simulink model "flightControlSystem2"  (R2019a)
settings: Solver=ode3  StartTime=0  StopTime=TFinal  FixedStep=Ts  RelTol=1e-3  EnableMultiTasking=on
InitFcn:
  | %生成模板
  | temp_Image = uint8(ones(120,160));
  | 
  | [m,n] = size(temp_Image);
  | angle = 10*pi/180;
  | 
  | left_point = 70;
  | right_point = 90;
  | j = 71;
  | for i = 1:50
  |     temp_left_point = floor(left_point - i*sin(angle));
  |     temp_right_point = floor(right_point + i*sin(angle));
  |     if temp_left_point < 1
  |         temp_left_point = 1;
  |     end
  |     if temp_right_point > 180
  |         temp_right_point = 180;
  |     end
  |     temp_Image(j,temp_left_point:temp_right_point) = 0;
  |     j = j+1;
  | end
undefined symbols (not defined in the file): codertarget, Controller, DiscIntNeverNeededParam, Discrete, Estimator, g, gray, init, pos_ref, Sensors, takeoff_flag, Time, Ts, Vehicle
libraries: simulink x60, visiontransforms x4, sharedtransform x3, ctrlSharedLib x2, visionsinks x2, sharedutil x1, visionanalysis x1, parrotlib x1
(part 1 of 3)
settings Model: ExtModeTrigDuration=80  Creator=The MathWorks, Inc.  LastModifiedBy=Sharlene
settings DataIOCC: LimitDataPoints=on  SaveFormat=StructureWithTime  SaveOutput=off  DSMLogging=off  SaveTime=off  ReturnWorkspaceOutputs=off
settings OptimizationCC: BlockReduction=off  EnhancedBackFolding=on  PassReuseOutputArgsAs=Individual arguments  MaxStackSize=64  OptimizeBlockOrder=speed  DifferentSizesBufferReuse=on  OptimizationCustomize=off
settings DebuggingCC: AlgebraicLoopMsg=none  ParameterPrecisionLossMsg=none  ParameterTunabilityLossMsg=error  UnconnectedInputMsg=none  UnconnectedOutputMsg=none  UnconnectedLineMsg=none  BusObjectLabelMismatch=error  PregeneratedLibrarySubsystemCodeDiagnostic=none  SFUnexpectedBacktrackingDiag=warning  SFNoUnconditionalDefaultTransitionDiag=warning  SFExecutionAtInitializationDiag=none  ArithmeticOperatorsInVariantConditions=warning
settings HardwareCC: ProdBitPerPointer=32  ProdBitPerSizeT=32  ProdBitPerPtrDiffT=32  ProdLargestAtomicInteger=Long  ProdWordSize=32  ProdHWDeviceType=ARM Compatible->ARM 9  UseEmbeddedCoderFeatures=off  UseSimulinkCoderFeatures=off
settings ModelReferenceCC: ModelReferenceNumInstancesAllowed=Single  PropagateSignalLabelsOutOfModel=off
settings SFSimCC: SimUseLocalCustomCode=off  MATLABDynamicMemAlloc=off
settings RTWCC: SystemTargetFile=ert.tlc  HardwareBoard=PARROT Mambo  TLCOptions=-aInlineSetEventsForThisBaseRateFcn=TLC_FALSE -aSuppressMultiTaskScheduler=TLC_FALSE -aRateBasedStepFcn=1  TemplateMakefile=ert_default_tmf  RTWUseLocalCustomCode=off  Toolchain=Sourcery G++ Lite GNU Toolchain for Drones  IncludeHyperlinkInReport=on
settings CodeAppCC: ForceParamTrailComments=on  IgnoreCustomStorageClasses=off  MaxIdLength=63  OperatorAnnotations=on  SimulinkDataObjDesc=on  SFDataObjDesc=on  InsertBlockDesc=on
settings ERTTargetCC: CombineOutputUpdateFcns=off  SupportNonInlinedSFcns=on
settings ConfigComp: CovMetricSettings=dw  CovHtmlReporting=on  CovSaveCumulativeToWorkspaceVar=on  CovSaveSingleToWorkspaceVar=on  CovExternalEMLEnable=off  CovSFcnEnable=off

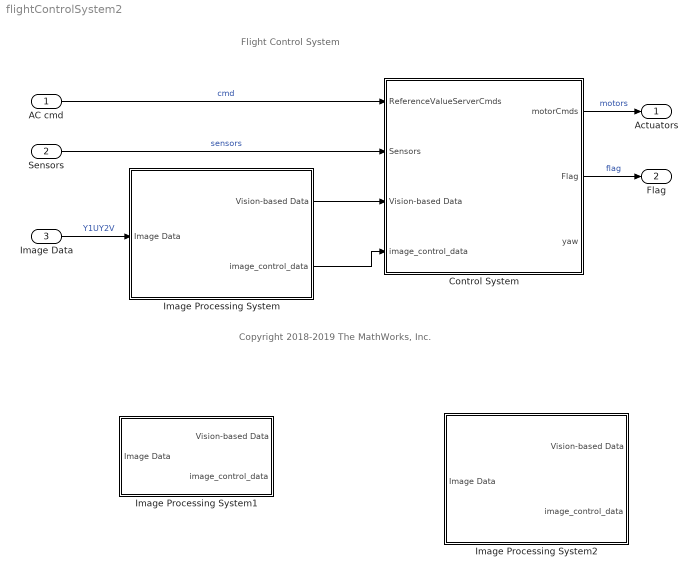
== system flightControlSystem2 ==
  note: Copyright 2018-2019 The MathWorks, Inc.
  note: Flight Control System
  AC cmd : Inport  OutDataTypeStr=Bus: CommandBus  BusOutputAsStruct=on
  Sensors : Inport  Port=2  OutDataTypeStr=Bus: SensorsBus  BusOutputAsStruct=on
  Image Data : Inport  Tag=IP_IN  InitFcn=codertarget.parrot.internal.inportCallback(gcb);  Port=3  OutDataTypeStr=uint8  PortDimensions=[4 9600]  BusOutputAsStruct=on
  Control System : Subsystem  InitFcn=codertarget.parrot.internal.fcsSubsystemCallback(gcb);  TreatAsAtomicUnit=on  SystemSampleTime=Ts
  Image Processing System : Subsystem  Tag=IP_SUB  InitFcn=codertarget.parrot.internal.ipSubsystemCallback(gcb);  TreatAsAtomicUnit=on  SystemSampleTime=40*Ts  RTWFcnName=ImageFunction
      settings: RTWSystemCode=Inline  RTWFcnNameOpts=User specified
  Image Processing System1 : Subsystem  Tag=IP_SUB  InitFcn=codertarget.parrot.internal.ipSubsystemCallback(gcb);  TreatAsAtomicUnit=on  SystemSampleTime=40*Ts  RTWFcnName=ImageFunction
      settings: RTWSystemCode=Inline  RTWFcnNameOpts=User specified
  Image Processing System2 : Subsystem  Tag=IP_SUB  InitFcn=codertarget.parrot.internal.ipSubsystemCallback(gcb);  TreatAsAtomicUnit=on  SystemSampleTime=40*Ts  RTWFcnName=ImageFunction
      settings: RTWSystemCode=Inline  RTWFcnNameOpts=User specified
  Actuators : Outport  OutDataTypeStr=single  PortDimensions=4
  Flag : Outport  Port=2  OutDataTypeStr=uint8  PortDimensions=1
  wires:
  AC cmd/1 -> Control System/1(ReferenceValueServerCmds)  "cmd"
  Control System/1(motorCmds) -> Actuators/1  "motors"
  Sensors/1 -> Control System/2(Sensors)  "sensors"
  Control System/2(Flag) -> Flag/1  "flag"
  Image Data/1 -> Image Processing System/1(Image Data)  "Y1UY2V"
  Image Processing System/1(Vision-based Data) -> Control System/3(Vision-based Data)
  Image Processing System/2(image_control_data) -> Control System/4("image_control_data ")

== system flightControlSystem2/Control System ==
  note: Position or Orientation Control
  note: Use this subsystem to change the path of the
      | Minidrone depending on the input Vision-based
      | Data
  note: Derived from the work by Sertac
      | Karaman and Fabian Riether
  ReferenceValueServerCmds : Inport  OutDataTypeStr=Bus: CommandBus
  Sensors : Inport  Port=2  OutDataTypeStr=Bus: SensorsBus  BusOutputAsStruct=on
  Vision-based Data : Inport  Port=3
  "image_control_data " : Inport  Port=4
  Bus Selector1 : BusSelector  OutputSignals=opticalFlow_data
  Bus Selector4 : BusSelector  OutputSignals=VisionSensors,SensorCalibration
  Control Mode Update : BusAssignment  AssignedSignals=controlModePosVSOrient
  Controller : Subsystem
  Crash Predictor Flags : Subsystem
  Path Planning : Subsystem
  Path Planning1 : Subsystem
  Path Planning2 : Subsystem
  State Estimator : Subsystem
  To Workspace : ToWorkspace  VariableName=estimatedStates  SaveFormat=Structure With Time  SampleTime=-1
  controlModePosVsOrient : Constant  OutDataTypeStr=boolean
  motorCmds : Outport
  Flag : Outport  Port=2
  yaw : Outport  Port=3
  wires:
  ReferenceValueServerCmds/1 -> Control Mode Update/1
  Bus Selector1/1 -> State Estimator/3(opticalFlow_datin)  "<opticalFlow_data>"
  Bus Selector4/2 -> State Estimator/4(sensorCalibration_datin)  "<SensorCalibration>"
  Path Planning/1(UpdatedReferenceCmds) -> Controller/1(ReferenceValueServerBus)
  Bus Selector4/1 -> Bus Selector1/1  "<VisionSensors>"
  Vision-based Data/1 -> Path Planning/3(drone_xyz)
  Crash Predictor Flags/1(Flag) -> Flag/1
  Control Mode Update/1 -> Path Planning/1(ReferenceValueServerCmds)
  controlModePosVsOrient/1 -> Control Mode Update/2, State Estimator/1(controlModePosVSOrient_flagin)
  Controller/1(motors_refout) -> motorCmds/1
  Sensors/1 -> State Estimator/2(sensor_data_in), Crash Predictor Flags/3(Sensors), Bus Selector4/1
  State Estimator/1(states_estim) -> Crash Predictor Flags/1(states_estim), To Workspace/1, Controller/2(states_estim)
  State Estimator/2(Alt_prs) -> Crash Predictor Flags/2(Alt_prs)
  Controller/2(yaw) -> Path Planning/4(yaw), yaw/1
  "image_control_data "/1 -> Path Planning/2(image_control_data)

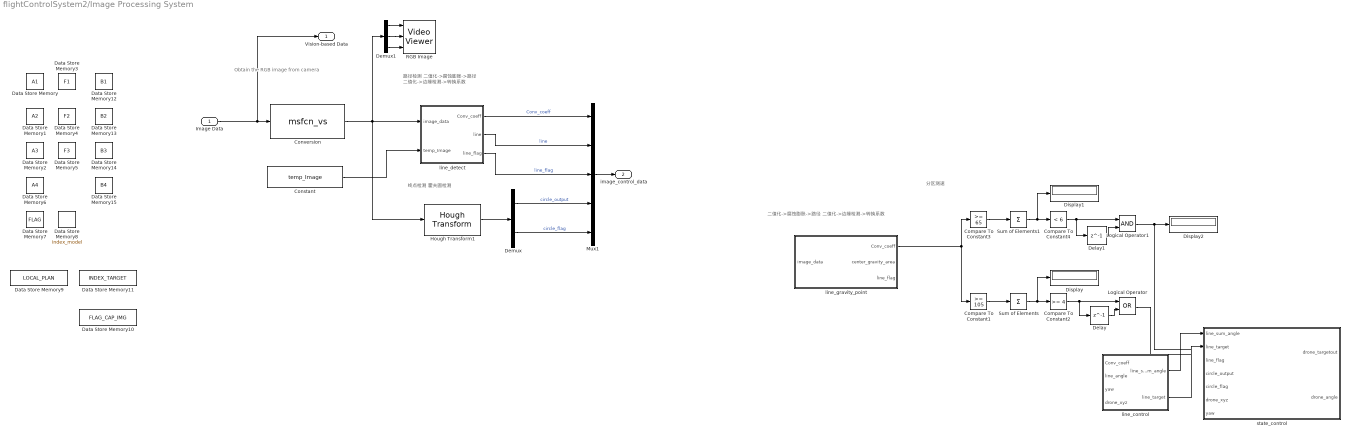
== system flightControlSystem2/Image Processing System ==
  note: 二值化->腐蚀膨胀->路径
      | 二值化->边缘检测->转换系数
  note: 终点检测
      | 霍夫圆检测
  note: Obtain the RGB image from camera
  note: 路径检测
      | 二值化->腐蚀膨胀->路径
      | 二值化->边缘检测->转换系数
  note: 分区测速
  Image Data : Inport
  Compare To Constant1 : simulink/Logic and Bit Operations/Compare To Constant  relop=>=  const=105  OutDataTypeStr=boolean
  Compare To Constant2 : simulink/Logic and Bit Operations/Compare To Constant  relop=>=  const=4  OutDataTypeStr=boolean
  Compare To Constant3 : simulink/Logic and Bit Operations/Compare To Constant  relop=>=  const=65  OutDataTypeStr=boolean
  Compare To Constant4 : simulink/Logic and Bit Operations/Compare To Constant  relop=<  const=6  OutDataTypeStr=boolean
  Constant : Constant  Value=temp_Image
  Conversion : M-S-Function  FunctionName=msfcn_vs
      mask Display: disp('PARROT Image Conversion')
  Data Store Memory : DataStoreMemory  DataStoreName=A1  ReadBeforeWriteMsg=warning  WriteAfterWriteMsg=warning  WriteAfterReadMsg=warning  ShowAdditionalParam=off  OutDataTypeStr=double
  Data Store Memory1 : DataStoreMemory  DataStoreName=A2  ReadBeforeWriteMsg=warning  WriteAfterWriteMsg=warning  WriteAfterReadMsg=warning  ShowAdditionalParam=off  OutDataTypeStr=double
  Data Store Memory10 : DataStoreMemory  DataStoreName=FLAG_CAP_IMG  ReadBeforeWriteMsg=warning  WriteAfterWriteMsg=warning  WriteAfterReadMsg=warning  InitialValue=1  ShowAdditionalParam=off  OutDataTypeStr=double
  Data Store Memory11 : DataStoreMemory  DataStoreName=INDEX_TARGET  ReadBeforeWriteMsg=warning  WriteAfterWriteMsg=warning  WriteAfterReadMsg=warning  InitialValue=1  ShowAdditionalParam=off  OutDataTypeStr=double
  Data Store Memory12 : DataStoreMemory  DataStoreName=B1  ReadBeforeWriteMsg=warning  WriteAfterWriteMsg=warning  WriteAfterReadMsg=warning  ShowAdditionalParam=off  OutDataTypeStr=double
  Data Store Memory13 : DataStoreMemory  DataStoreName=B2  ReadBeforeWriteMsg=warning  WriteAfterWriteMsg=warning  WriteAfterReadMsg=warning  ShowAdditionalParam=off  OutDataTypeStr=double
  Data Store Memory14 : DataStoreMemory  DataStoreName=B3  ReadBeforeWriteMsg=warning  WriteAfterWriteMsg=warning  WriteAfterReadMsg=warning  ShowAdditionalParam=off  OutDataTypeStr=double
  Data Store Memory15 : DataStoreMemory  DataStoreName=B4  ReadBeforeWriteMsg=warning  WriteAfterWriteMsg=warning  WriteAfterReadMsg=warning  ShowAdditionalParam=off  OutDataTypeStr=double
  Data Store Memory2 : DataStoreMemory  DataStoreName=A3  ReadBeforeWriteMsg=warning  WriteAfterWriteMsg=warning  WriteAfterReadMsg=warning  ShowAdditionalParam=off  OutDataTypeStr=double
  Data Store Memory3 : DataStoreMemory  DataStoreName=F1  ReadBeforeWriteMsg=warning  WriteAfterWriteMsg=warning  WriteAfterReadMsg=warning  ShowAdditionalParam=off  OutDataTypeStr=double
  Data Store Memory4 : DataStoreMemory  DataStoreName=F2  ReadBeforeWriteMsg=warning  WriteAfterWriteMsg=warning  WriteAfterReadMsg=warning  ShowAdditionalParam=off  OutDataTypeStr=double
  Data Store Memory5 : DataStoreMemory  DataStoreName=F3  ReadBeforeWriteMsg=warning  WriteAfterWriteMsg=warning  WriteAfterReadMsg=warning  InitialValue=[0;0;0]  ShowAdditionalParam=off  OutDataTypeStr=double
  Data Store Memory6 : DataStoreMemory  DataStoreName=A4  ReadBeforeWriteMsg=warning  WriteAfterWriteMsg=warning  WriteAfterReadMsg=warning  ShowAdditionalParam=off  OutDataTypeStr=double
  Data Store Memory7 : DataStoreMemory  DataStoreName=FLAG  ReadBeforeWriteMsg=warning  WriteAfterWriteMsg=warning  WriteAfterReadMsg=warning  ShowAdditionalParam=off  OutDataTypeStr=double
  Data Store Memory8 : DataStoreMemory  DataStoreName=index_model  ReadBeforeWriteMsg=warning  WriteAfterWriteMsg=warning  WriteAfterReadMsg=warning  InitialValue=1  ShowAdditionalParam=off  OutDataTypeStr=double
  Data Store Memory9 : DataStoreMemory  DataStoreName=LOCAL_PLAN  ReadBeforeWriteMsg=warning  WriteAfterWriteMsg=warning  WriteAfterReadMsg=warning  InitialValue=ones(10,2)  ShowAdditionalParam=off  OutDataTypeStr=double
  Delay : Delay  DelayLength=1  InitialCondition=0
  Delay1 : Delay  DelayLength=1  InitialCondition=0
  Demux : Demux  Outputs=2
  Demux1 : Demux  Outputs=3
  Display : Display
  Display1 : Display
  Display2 : Display
  Hough Transform1 : visiontransforms/Hough Transform  theta_res=pi/180  rho_res=1  out_theta_rho=off  outdtmode=double  roundingMode=Nearest  overflowMode=on  firstCoeffMode=Binary point scaling  firstCoeffWordLength=16  firstCoeffFracLength=14  firstCoeffSlope=2^-14  secondCoeffMode=Binary point scaling  secondCoeffWordLength=32  secondCoeffFracLength=16  secondCoeffSlope=2^-16  prodOutputMode=Binary point scaling  prodOutputWordLength=32  prodOutputFracLength=20  prodOutputSlope=2^-20  accumMode=Binary point scaling  accumWordLength=32  accumFracLength=20  accumSlope=2^-20  outputMode=Binary point scaling  outputWordLength=16  outputFracLength=0  outputSlope=2^0  memoryMode=Binary point scaling  memoryWordLength=32  memoryFracLength=16  memorySlope=2^-16
      settings: SourceProductName=Computer Vision Toolbox  SourceProductBaseCode=VP
  Logical Operator : Logic  Operator=OR  AllPortsSameDT=off  OutDataTypeStr=boolean
  Logical Operator1 : Logic  AllPortsSameDT=off  OutDataTypeStr=boolean
  Mux1 : Mux  Inputs=5
  RGB Image : VideoViewer  imagePorts=separate color signals  FigPos=[238 767 414 175]
  Sum of Elements : Sum  Inputs=+  OutDataTypeStr=int8
  Sum of Elements1 : Sum  Inputs=+  OutDataTypeStr=int8
  line_control : MATLAB Function  TreatAsAtomicUnit=on
  line_detect : MATLAB Function  TreatAsAtomicUnit=on
  line_gravity_point : MATLAB Function  TreatAsAtomicUnit=on
  state_control : MATLAB Function  TreatAsAtomicUnit=on
  Vision-based Data : Outport
  image_control_data : Outport  Port=2
  wires:
  Image Data/1 -> Vision-based Data/1, Conversion/1
  Constant/1 -> line_detect/2(temp_Image)
  line_control/1(line_sum_angle) -> state_control/1(line_sum_angle)
  line_control/2(line_target) -> state_control/2(line_target)
  Sum of Elements1/1 -> Compare To Constant4/1, Display1/1
  Compare To Constant4/1 -> Delay1/1, Logical Operator1/1
  Compare To Constant3/1 -> Sum of Elements1/1
  Delay/1 -> Logical Operator/2
  Compare To Constant2/1 -> Logical Operator/1, Delay/1
  Logical Operator1/1 -> Display2/1
  Sum of Elements/1 -> Compare To Constant2/1, Display/1
  line_gravity_point/1(Conv_coeff) -> Compare To Constant1/1, Compare To Constant3/1
  Logical Operator/1 -> ?
  Compare To Constant1/1 -> Sum of Elements/1
  Delay1/1 -> Logical Operator1/2
  Conversion/1 -> line_detect/1(image_data), Hough Transform1/1, Demux1/1
  Demux/1 -> Mux1/4  "circle_output"
  line_detect/3(line_flag) -> Mux1/3  "line_flag"
  line_detect/1(Conv_coeff) -> Mux1/1  "Conv_coeff"
  Mux1/1 -> image_control_data/1
  Demux/2 -> Mux1/5  "circle_flag"
  Hough Transform1/1 -> Demux/1
  line_detect/2(line) -> Mux1/2  "line"
  Demux1/1 -> RGB Image/1
  Demux1/2 -> RGB Image/2
  Demux1/3 -> RGB Image/3

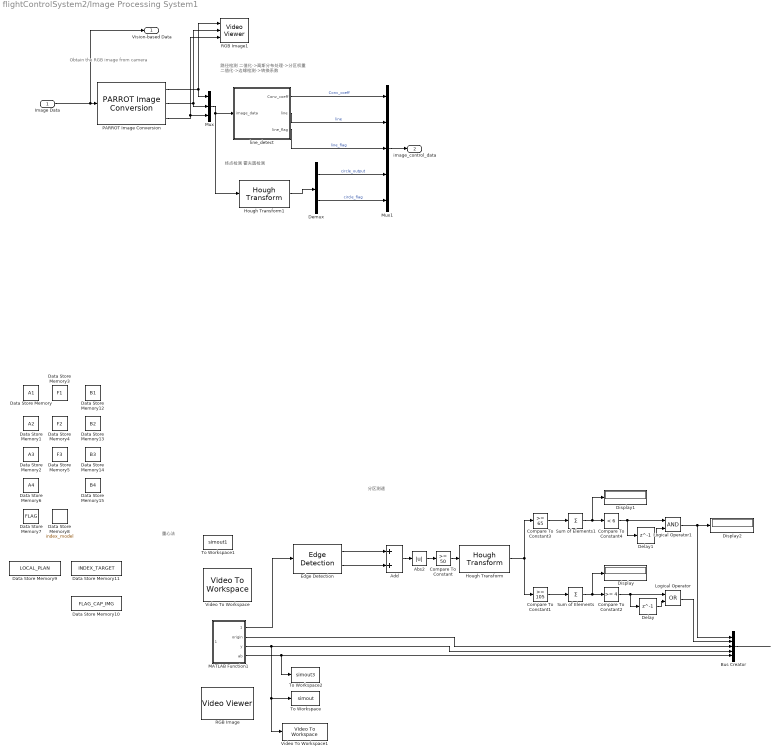
== system flightControlSystem2/Image Processing System1 ==
  note: 分区测速
  note: 重心法
  note: 路径检测
      | 二值化->高斯分布处理->分区权重
      | 二值化->边缘检测->转换系数
  note: 终点检测
      | 霍夫圆检测
  note: Obtain the RGB image from camera
  Image Data : Inport
  Abs2 : Abs
  Add : Sum
  Bus Creator : BusCreator  Inputs=5
  Compare To Constant : simulink/Logic and Bit Operations/Compare To Constant  relop=>=  const=50  OutDataTypeStr=boolean
  Compare To Constant1 : simulink/Logic and Bit Operations/Compare To Constant  relop=>=  const=105  OutDataTypeStr=boolean
  Compare To Constant2 : simulink/Logic and Bit Operations/Compare To Constant  relop=>=  const=4  OutDataTypeStr=boolean
  Compare To Constant3 : simulink/Logic and Bit Operations/Compare To Constant  relop=>=  const=65  OutDataTypeStr=boolean
  Compare To Constant4 : simulink/Logic and Bit Operations/Compare To Constant  relop=<  const=6  OutDataTypeStr=boolean
  Data Store Memory : DataStoreMemory  DataStoreName=A1  ReadBeforeWriteMsg=warning  WriteAfterWriteMsg=warning  WriteAfterReadMsg=warning  ShowAdditionalParam=off  OutDataTypeStr=double
  Data Store Memory1 : DataStoreMemory  DataStoreName=A2  ReadBeforeWriteMsg=warning  WriteAfterWriteMsg=warning  WriteAfterReadMsg=warning  ShowAdditionalParam=off  OutDataTypeStr=double
  Data Store Memory10 : DataStoreMemory  DataStoreName=FLAG_CAP_IMG  ReadBeforeWriteMsg=warning  WriteAfterWriteMsg=warning  WriteAfterReadMsg=warning  InitialValue=1  ShowAdditionalParam=off  OutDataTypeStr=double
  Data Store Memory11 : DataStoreMemory  DataStoreName=INDEX_TARGET  ReadBeforeWriteMsg=warning  WriteAfterWriteMsg=warning  WriteAfterReadMsg=warning  InitialValue=1  ShowAdditionalParam=off  OutDataTypeStr=double
  Data Store Memory12 : DataStoreMemory  DataStoreName=B1  ReadBeforeWriteMsg=warning  WriteAfterWriteMsg=warning  WriteAfterReadMsg=warning  ShowAdditionalParam=off  OutDataTypeStr=double
  Data Store Memory13 : DataStoreMemory  DataStoreName=B2  ReadBeforeWriteMsg=warning  WriteAfterWriteMsg=warning  WriteAfterReadMsg=warning  ShowAdditionalParam=off  OutDataTypeStr=double
  Data Store Memory14 : DataStoreMemory  DataStoreName=B3  ReadBeforeWriteMsg=warning  WriteAfterWriteMsg=warning  WriteAfterReadMsg=warning  ShowAdditionalParam=off  OutDataTypeStr=double
  Data Store Memory15 : DataStoreMemory  DataStoreName=B4  ReadBeforeWriteMsg=warning  WriteAfterWriteMsg=warning  WriteAfterReadMsg=warning  ShowAdditionalParam=off  OutDataTypeStr=double
  Data Store Memory2 : DataStoreMemory  DataStoreName=A3  ReadBeforeWriteMsg=warning  WriteAfterWriteMsg=warning  WriteAfterReadMsg=warning  ShowAdditionalParam=off  OutDataTypeStr=double
  Data Store Memory3 : DataStoreMemory  DataStoreName=F1  ReadBeforeWriteMsg=warning  WriteAfterWriteMsg=warning  WriteAfterReadMsg=warning  ShowAdditionalParam=off  OutDataTypeStr=double
  Data Store Memory4 : DataStoreMemory  DataStoreName=F2  ReadBeforeWriteMsg=warning  WriteAfterWriteMsg=warning  WriteAfterReadMsg=warning  ShowAdditionalParam=off  OutDataTypeStr=double
  Data Store Memory5 : DataStoreMemory  DataStoreName=F3  ReadBeforeWriteMsg=warning  WriteAfterWriteMsg=warning  WriteAfterReadMsg=warning  InitialValue=[0;0;0]  ShowAdditionalParam=off  OutDataTypeStr=double
  Data Store Memory6 : DataStoreMemory  DataStoreName=A4  ReadBeforeWriteMsg=warning  WriteAfterWriteMsg=warning  WriteAfterReadMsg=warning  ShowAdditionalParam=off  OutDataTypeStr=double
  Data Store Memory7 : DataStoreMemory  DataStoreName=FLAG  ReadBeforeWriteMsg=warning  WriteAfterWriteMsg=warning  WriteAfterReadMsg=warning  ShowAdditionalParam=off  OutDataTypeStr=double
  Data Store Memory8 : DataStoreMemory  DataStoreName=index_model  ReadBeforeWriteMsg=warning  WriteAfterWriteMsg=warning  WriteAfterReadMsg=warning  InitialValue=1  ShowAdditionalParam=off  OutDataTypeStr=double
  Data Store Memory9 : DataStoreMemory  DataStoreName=LOCAL_PLAN  ReadBeforeWriteMsg=warning  WriteAfterWriteMsg=warning  WriteAfterReadMsg=warning  InitialValue=ones(10,2)  ShowAdditionalParam=off  OutDataTypeStr=double
  Delay : Delay  DelayLength=1  InitialCondition=0
  Delay1 : Delay  DelayLength=1  InitialCondition=0
  Demux : Demux  Outputs=2
  Display : Display
  Display1 : Display
  Display2 : Display
  Edge Detection : visionanalysis/Edge Detection  method=Sobel  outputType=Gradient components  userDefinedThreshold=off  thresholdSource=Input port  threshold=20  thresholdTuning=4  edgeThinning=off  threshold_canny=[0.25 0.60]  autoPercent=70  sigma=1  roundingMode=Floor  overflowMode=off  prodOutputMode=Binary point scaling  prodOutputWordLength=32  prodOutputFracLength=8  prodOutputSlope=2^-8  accumSlope=2^-8  outputSlope=2^-4
      settings: SourceProductName=Computer Vision Toolbox  SourceProductBaseCode=VP
  Hough Transform : visiontransforms/Hough Transform  theta_res=pi/180  rho_res=1  out_theta_rho=off  outdtmode=double  roundingMode=Nearest  overflowMode=on  firstCoeffMode=Binary point scaling  firstCoeffWordLength=16  firstCoeffFracLength=14  firstCoeffSlope=2^-14  secondCoeffMode=Binary point scaling  secondCoeffWordLength=32  secondCoeffFracLength=16  secondCoeffSlope=2^-16  prodOutputMode=Binary point scaling  prodOutputWordLength=32  prodOutputFracLength=20  prodOutputSlope=2^-20  accumMode=Binary point scaling  accumWordLength=32  accumFracLength=20  accumSlope=2^-20  outputMode=Binary point scaling  outputWordLength=16  outputFracLength=0  outputSlope=2^0  memoryMode=Binary point scaling  memoryWordLength=32  memoryFracLength=16  memorySlope=2^-16
      settings: SourceProductName=Computer Vision Toolbox  SourceProductBaseCode=VP
  Hough Transform1 : visiontransforms/Hough Transform  theta_res=pi/180  rho_res=1  out_theta_rho=off  outdtmode=double  roundingMode=Nearest  overflowMode=on  firstCoeffMode=Binary point scaling  firstCoeffWordLength=16  firstCoeffFracLength=14  firstCoeffSlope=2^-14  secondCoeffMode=Binary point scaling  secondCoeffWordLength=32  secondCoeffFracLength=16  secondCoeffSlope=2^-16  prodOutputMode=Binary point scaling  prodOutputWordLength=32  prodOutputFracLength=20  prodOutputSlope=2^-20  accumMode=Binary point scaling  accumWordLength=32  accumFracLength=20  accumSlope=2^-20  outputMode=Binary point scaling  outputWordLength=16  outputFracLength=0  outputSlope=2^0  memoryMode=Binary point scaling  memoryWordLength=32  memoryFracLength=16  memorySlope=2^-16
      settings: SourceProductName=Computer Vision Toolbox  SourceProductBaseCode=VP
  Logical Operator : Logic  Operator=OR  AllPortsSameDT=off  OutDataTypeStr=boolean
  Logical Operator1 : Logic  AllPortsSameDT=off  OutDataTypeStr=boolean
  MATLAB Function1 : MATLAB Function  TreatAsAtomicUnit=on
  Mux : Mux  Inputs=3
  Mux1 : Mux  Inputs=5
  PARROT Image Conversion : parrotlib/PARROT Image Conversion  ImageFormat=RGB  R=on  Y=on  G=on  U=on  B=on  V=on
      settings: SourceProductName=Simulink Support Package for PARROT Minidrones
  RGB Image : VideoViewer  imagePorts=separate color signals  colormapValue=gray(256)  FigPos=[980.636363636364 356.545454545455 317.090909090909 234.909090909091]
  RGB Image1 : VideoViewer  imagePorts=separate color signals  FigPos=[238 767 414 175]
  Sum of Elements : Sum  Inputs=+  OutDataTypeStr=int8
  Sum of Elements1 : Sum  Inputs=+  OutDataTypeStr=int8
  To Workspace : ToWorkspace  VariableName=simout  SaveFormat=Timeseries  SampleTime=-1
  To Workspace1 : ToWorkspace  VariableName=simout1  SaveFormat=Timeseries  SampleTime=-1
  To Workspace2 : ToWorkspace  VariableName=simout3  SaveFormat=Timeseries  SampleTime=-1
  Video To Workspace : visionsinks/Video To Workspace  VariableName=RI  NumInputs=1  DataLimit=1  DecimationFactor=1  LogFi=off  InPortLabels=R|G|B
      settings: SourceProductName=Computer Vision Toolbox  SourceProductBaseCode=VP
  Video To Workspace1 : visionsinks/Video To Workspace  VariableName=RI2  NumInputs=1  DataLimit=1  DecimationFactor=1  LogFi=off  InPortLabels=R|G|B
      settings: SourceProductName=Computer Vision Toolbox  SourceProductBaseCode=VP
  line_detect : MATLAB Function  TreatAsAtomicUnit=on
  Vision-based Data : Outport
  image_control_data : Outport  Port=2
  wires:
  ? -> MATLAB Function1/1(R_Matrix), To Workspace1/1, Video To Workspace/1, RGB Image/1
  Sum of Elements1/1 -> Compare To Constant4/1, Display1/1
  Compare To Constant4/1 -> Delay1/1, Logical Operator1/1
  Compare To Constant3/1 -> Sum of Elements1/1
  Delay/1 -> Logical Operator/2
  Edge Detection/2 -> Add/2
  MATLAB Function1/1(R_stright) -> Edge Detection/1
  Compare To Constant2/1 -> Logical Operator/1, Delay/1
  Logical Operator1/1 -> Bus Creator/1, Display2/1
  Sum of Elements/1 -> Compare To Constant2/1, Display/1
  Compare To Constant1/1 -> Sum of Elements/1
  Edge Detection/1 -> Add/1
  Abs2/1 -> Compare To Constant/1
  Add/1 -> Abs2/1
  ? -> RGB Image/2
  ? -> RGB Image/3
  Bus Creator/1 -> ?
  MATLAB Function1/2(origin) -> Bus Creator/3
  MATLAB Function1/3(y) -> Bus Creator/4, To Workspace/1, Video To Workspace1/1
  Hough Transform/1 -> Compare To Constant1/1, Compare To Constant3/1
  MATLAB Function1/4(ab) -> Bus Creator/5, To Workspace2/1
  Compare To Constant/1 -> Hough Transform/1
  Logical Operator/1 -> Bus Creator/2
  Delay1/1 -> Logical Operator1/2
  Hough Transform1/1 -> Demux/1
  Demux/2 -> Mux1/5  "circle_flag"
  Image Data/1 -> Vision-based Data/1, PARROT Image Conversion/1
  PARROT Image Conversion/2 -> RGB Image1/2, Mux/2
  PARROT Image Conversion/3 -> RGB Image1/3, Mux/3
  line_detect/2(line) -> Mux1/2  "line"
  line_detect/1(Conv_coeff) -> Mux1/1  "Conv_coeff"
  line_detect/3(line_flag) -> Mux1/3  "line_flag"
  PARROT Image Conversion/1 -> RGB Image1/1, Mux/1
  Demux/1 -> Mux1/4  "circle_output"
  Mux/1 -> Hough Transform1/1, line_detect/1(image_data)
  Mux1/1 -> image_control_data/1

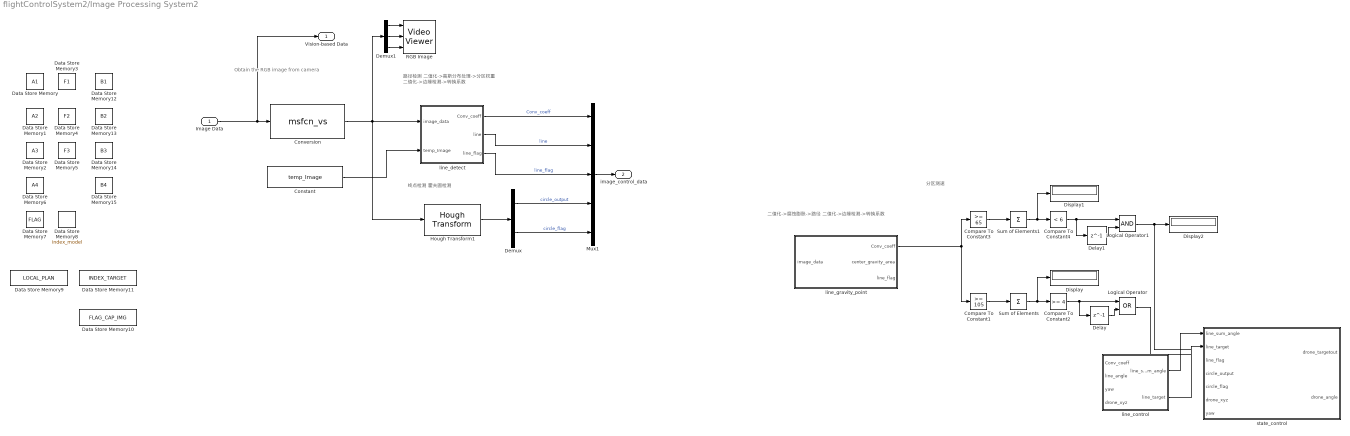
== system flightControlSystem2/Image Processing System2 ==
  note: 二值化->腐蚀膨胀->路径
      | 二值化->边缘检测->转换系数
  note: 终点检测
      | 霍夫圆检测
  note: Obtain the RGB image from camera
  note: 路径检测
      | 二值化->高斯分布处理->分区权重
      | 二值化->边缘检测->转换系数
  note: 分区测速
  Image Data : Inport
  Compare To Constant1 : simulink/Logic and Bit Operations/Compare To Constant  relop=>=  const=105  OutDataTypeStr=boolean
  Compare To Constant2 : simulink/Logic and Bit Operations/Compare To Constant  relop=>=  const=4  OutDataTypeStr=boolean
  Compare To Constant3 : simulink/Logic and Bit Operations/Compare To Constant  relop=>=  const=65  OutDataTypeStr=boolean
  Compare To Constant4 : simulink/Logic and Bit Operations/Compare To Constant  relop=<  const=6  OutDataTypeStr=boolean
  Constant : Constant  Value=temp_Image
  Conversion : M-S-Function  FunctionName=msfcn_vs
      mask Display: disp('PARROT Image Conversion')
  Data Store Memory : DataStoreMemory  DataStoreName=A1  ReadBeforeWriteMsg=warning  WriteAfterWriteMsg=warning  WriteAfterReadMsg=warning  ShowAdditionalParam=off  OutDataTypeStr=double
  Data Store Memory1 : DataStoreMemory  DataStoreName=A2  ReadBeforeWriteMsg=warning  WriteAfterWriteMsg=warning  WriteAfterReadMsg=warning  ShowAdditionalParam=off  OutDataTypeStr=double
  Data Store Memory10 : DataStoreMemory  DataStoreName=FLAG_CAP_IMG  ReadBeforeWriteMsg=warning  WriteAfterWriteMsg=warning  WriteAfterReadMsg=warning  InitialValue=1  ShowAdditionalParam=off  OutDataTypeStr=double
  Data Store Memory11 : DataStoreMemory  DataStoreName=INDEX_TARGET  ReadBeforeWriteMsg=warning  WriteAfterWriteMsg=warning  WriteAfterReadMsg=warning  InitialValue=1  ShowAdditionalParam=off  OutDataTypeStr=double
  Data Store Memory12 : DataStoreMemory  DataStoreName=B1  ReadBeforeWriteMsg=warning  WriteAfterWriteMsg=warning  WriteAfterReadMsg=warning  ShowAdditionalParam=off  OutDataTypeStr=double
  Data Store Memory13 : DataStoreMemory  DataStoreName=B2  ReadBeforeWriteMsg=warning  WriteAfterWriteMsg=warning  WriteAfterReadMsg=warning  ShowAdditionalParam=off  OutDataTypeStr=double
  Data Store Memory14 : DataStoreMemory  DataStoreName=B3  ReadBeforeWriteMsg=warning  WriteAfterWriteMsg=warning  WriteAfterReadMsg=warning  ShowAdditionalParam=off  OutDataTypeStr=double
  Data Store Memory15 : DataStoreMemory  DataStoreName=B4  ReadBeforeWriteMsg=warning  WriteAfterWriteMsg=warning  WriteAfterReadMsg=warning  ShowAdditionalParam=off  OutDataTypeStr=double
  Data Store Memory2 : DataStoreMemory  DataStoreName=A3  ReadBeforeWriteMsg=warning  WriteAfterWriteMsg=warning  WriteAfterReadMsg=warning  ShowAdditionalParam=off  OutDataTypeStr=double
  Data Store Memory3 : DataStoreMemory  DataStoreName=F1  ReadBeforeWriteMsg=warning  WriteAfterWriteMsg=warning  WriteAfterReadMsg=warning  ShowAdditionalParam=off  OutDataTypeStr=double
  Data Store Memory4 : DataStoreMemory  DataStoreName=F2  ReadBeforeWriteMsg=warning  WriteAfterWriteMsg=warning  WriteAfterReadMsg=warning  ShowAdditionalParam=off  OutDataTypeStr=double
  Data Store Memory5 : DataStoreMemory  DataStoreName=F3  ReadBeforeWriteMsg=warning  WriteAfterWriteMsg=warning  WriteAfterReadMsg=warning  InitialValue=[0;0;0]  ShowAdditionalParam=off  OutDataTypeStr=double
  Data Store Memory6 : DataStoreMemory  DataStoreName=A4  ReadBeforeWriteMsg=warning  WriteAfterWriteMsg=warning  WriteAfterReadMsg=warning  ShowAdditionalParam=off  OutDataTypeStr=double
  Data Store Memory7 : DataStoreMemory  DataStoreName=FLAG  ReadBeforeWriteMsg=warning  WriteAfterWriteMsg=warning  WriteAfterReadMsg=warning  ShowAdditionalParam=off  OutDataTypeStr=double
  Data Store Memory8 : DataStoreMemory  DataStoreName=index_model  ReadBeforeWriteMsg=warning  WriteAfterWriteMsg=warning  WriteAfterReadMsg=warning  InitialValue=1  ShowAdditionalParam=off  OutDataTypeStr=double
  Data Store Memory9 : DataStoreMemory  DataStoreName=LOCAL_PLAN  ReadBeforeWriteMsg=warning  WriteAfterWriteMsg=warning  WriteAfterReadMsg=warning  InitialValue=ones(10,2)  ShowAdditionalParam=off  OutDataTypeStr=double
  Delay : Delay  DelayLength=1  InitialCondition=0
  Delay1 : Delay  DelayLength=1  InitialCondition=0
  Demux : Demux  Outputs=2
  Demux1 : Demux  Outputs=3
  Display : Display
  Display1 : Display
  Display2 : Display
  Hough Transform1 : visiontransforms/Hough Transform  theta_res=pi/180  rho_res=1  out_theta_rho=off  outdtmode=double  roundingMode=Nearest  overflowMode=on  firstCoeffMode=Binary point scaling  firstCoeffWordLength=16  firstCoeffFracLength=14  firstCoeffSlope=2^-14  secondCoeffMode=Binary point scaling  secondCoeffWordLength=32  secondCoeffFracLength=16  secondCoeffSlope=2^-16  prodOutputMode=Binary point scaling  prodOutputWordLength=32  prodOutputFracLength=20  prodOutputSlope=2^-20  accumMode=Binary point scaling  accumWordLength=32  accumFracLength=20  accumSlope=2^-20  outputMode=Binary point scaling  outputWordLength=16  outputFracLength=0  outputSlope=2^0  memoryMode=Binary point scaling  memoryWordLength=32  memoryFracLength=16  memorySlope=2^-16
      settings: SourceProductName=Computer Vision Toolbox  SourceProductBaseCode=VP
  Logical Operator : Logic  Operator=OR  AllPortsSameDT=off  OutDataTypeStr=boolean
  Logical Operator1 : Logic  AllPortsSameDT=off  OutDataTypeStr=boolean
  Mux1 : Mux  Inputs=5
  RGB Image : VideoViewer  imagePorts=separate color signals  FigPos=[238 767 414 175]
  Sum of Elements : Sum  Inputs=+  OutDataTypeStr=int8
  Sum of Elements1 : Sum  Inputs=+  OutDataTypeStr=int8
  line_control : MATLAB Function  TreatAsAtomicUnit=on
  line_detect : MATLAB Function  TreatAsAtomicUnit=on
  line_gravity_point : MATLAB Function  TreatAsAtomicUnit=on
  state_control : MATLAB Function  TreatAsAtomicUnit=on
  Vision-based Data : Outport
  image_control_data : Outport  Port=2
  wires:
  Image Data/1 -> Vision-based Data/1, Conversion/1
  Constant/1 -> line_detect/2(temp_Image)
  line_control/1(line_sum_angle) -> state_control/1(line_sum_angle)
  line_control/2(line_target) -> state_control/2(line_target)
  Sum of Elements1/1 -> Compare To Constant4/1, Display1/1
  Compare To Constant4/1 -> Delay1/1, Logical Operator1/1
  Compare To Constant3/1 -> Sum of Elements1/1
  Delay/1 -> Logical Operator/2
  Compare To Constant2/1 -> Logical Operator/1, Delay/1
  Logical Operator1/1 -> Display2/1
  Sum of Elements/1 -> Compare To Constant2/1, Display/1
  line_gravity_point/1(Conv_coeff) -> Compare To Constant1/1, Compare To Constant3/1
  Logical Operator/1 -> ?
  Compare To Constant1/1 -> Sum of Elements/1
  Delay1/1 -> Logical Operator1/2
  Conversion/1 -> line_detect/1(image_data), Hough Transform1/1, Demux1/1
  Demux/1 -> Mux1/4  "circle_output"
  line_detect/3(line_flag) -> Mux1/3  "line_flag"
  line_detect/1(Conv_coeff) -> Mux1/1  "Conv_coeff"
  Mux1/1 -> image_control_data/1
  Demux/2 -> Mux1/5  "circle_flag"
  Hough Transform1/1 -> Demux/1
  line_detect/2(line) -> Mux1/2  "line"
  Demux1/1 -> RGB Image/1
  Demux1/2 -> RGB Image/2
  Demux1/3 -> RGB Image/3

== system flightControlSystem2/Control System/Controller ==
  In Bus Element1 : Inport  PortName=ReferenceValueServerBus  Element=controlModePosVSOrient
  In Bus Element : Inport  PortName=ReferenceValueServerBus  Element=pos_ref
  In Bus Element5 : Inport  PortName=ReferenceValueServerBus  Element=pos_ref
  In Bus Element2 : Inport  PortName=ReferenceValueServerBus  Element=orient_ref
  In Bus Element6 : Inport  PortName=ReferenceValueServerBus  Element=orient_ref
  In Bus Element3 : Inport  PortName=ReferenceValueServerBus  Element=takeoff_flag
  states_estim : Inport  Port=2
  Attitude : Subsystem
  ControlMixer : Subsystem
  Scope : Scope
  Selector : Selector  InputPortWidth=3  IndexOptions=Index vector (dialog)  Indices=3  OutputSizes=1
  Selector1 : Selector  InputPortWidth=3  IndexOptions=Index vector (dialog)  Indices=[1 2]  OutputSizes=1
  Selector2 : Selector  InputPortWidth=3  IndexOptions=Index vector (dialog)  Indices=[2 3]  OutputSizes=1
  Selector3 : Selector  InputPortWidth=3  IndexOptions=Index vector (dialog)  Indices=1  OutputSizes=1
  Switch_refAtt : Switch  Criteria=u2 > Threshold
  XY-to-reference-orientation : Subsystem
  Yaw : Subsystem
  gravity feedforward/equilibrium thrust : Subsystem
  states_estim1 : InportShadow  Port=2
  states_estim2 : InportShadow  Port=2
  states_estim3 : InportShadow  Port=2
  thrustsToMotorCommands : Subsystem
  motors_refout : Outport
  yaw : Outport  Port=2
  wires:
  thrustsToMotorCommands/1(motors_cmdout) -> motors_refout/1
  In Bus Element5/1 -> Selector/1
  Attitude/2(tau_roll) -> ControlMixer/2(tau_roll)
  states_estim3/1 -> XY-to-reference-orientation/2(states_estim)
  In Bus Element6/1 -> Selector2/1
  In Bus Element/1 -> Selector1/1
  ControlMixer/1(thrusts_refout) -> thrustsToMotorCommands/1(thrusts_refin)
  Selector2/1 -> Switch_refAtt/3
  Attitude/1(tau_pitch) -> ControlMixer/1(tau_pitch)
  gravity feedforward/equilibrium thrust/1(altitude_cmd) -> ControlMixer/4(totalThrust)
  Selector1/1 -> XY-to-reference-orientation/1(posXY)  "pos"
  states_estim1/1 -> gravity feedforward/equilibrium thrust/1(states_estim)
  Selector/1 -> gravity feedforward/equilibrium thrust/2(PosZ)
  Yaw/1(yaw) -> yaw/1, XY-to-reference-orientation/3(yaw)
  In Bus Element3/1 -> Scope/1, gravity feedforward/equilibrium thrust/3(takeoff_flag)
  states_estim/1 -> Yaw/2(states_estim)
  XY-to-reference-orientation/1(pitch_roll_cmd) -> Switch_refAtt/1
  In Bus Element2/1 -> Selector3/1
  Yaw/2(tau_yaw) -> ControlMixer/3(tau_yaw)
  In Bus Element1/1 -> Switch_refAtt/2
  Switch_refAtt/1 -> Attitude/1(refAttitude)
  states_estim2/1 -> Attitude/2(states_estim)

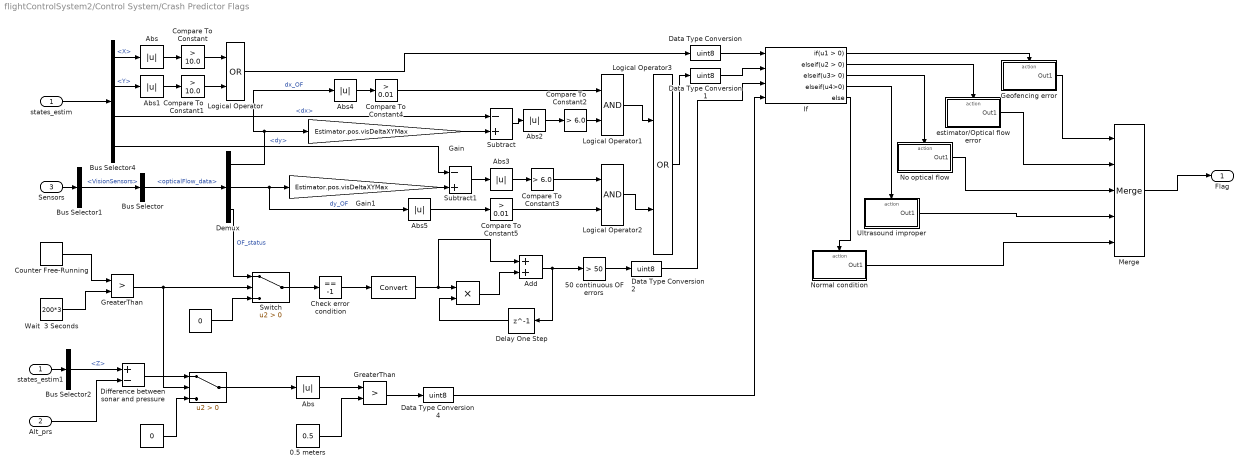
== system flightControlSystem2/Control System/Crash Predictor Flags ==
  states_estim : Inport
  Alt_prs : Inport  Port=2
  Sensors : Inport  Port=3
  " " : Constant  Value=0
  "  " : Product  Inputs=**
  "   " : DataTypeConversion
  "    " : Constant  Value=0  OutDataTypeStr=single
  "         " : Switch  Criteria=u2 > Threshold
  0.5 meters : Constant  Value=0.5
  "50 continuous OF errors " : simulink/Logic and Bit Operations/Compare To Constant  relop=>  const=50  OutDataTypeStr=boolean
  Abs{,1..5} (6 alike) : Abs
  "Abs  " : Abs
  Add : Sum
  Bus Selector : BusSelector  OutputSignals=opticalFlow_data
  Bus Selector1 : BusSelector  OutputSignals=VisionSensors
  Bus Selector2 : BusSelector  OutputSignals=Z
  Bus Selector4 : BusSelector  OutputSignals=X,Y,dx,dy
  Check error condition : simulink/Logic and Bit Operations/Compare To Constant  relop===  const=-1  OutDataTypeStr=boolean
  Compare To Constant : simulink/Logic and Bit Operations/Compare To Constant  relop=>  const=10.0  OutDataTypeStr=boolean
  Compare To Constant1 : simulink/Logic and Bit Operations/Compare To Constant  relop=>  const=10.0  OutDataTypeStr=boolean
  Compare To Constant2 : simulink/Logic and Bit Operations/Compare To Constant  relop=>  const=6.0  OutDataTypeStr=boolean
  Compare To Constant3 : simulink/Logic and Bit Operations/Compare To Constant  relop=>  const=6.0  OutDataTypeStr=boolean
  Compare To Constant4 : simulink/Logic and Bit Operations/Compare To Constant  relop=>  const=0.01  OutDataTypeStr=boolean
  Compare To Constant5 : simulink/Logic and Bit Operations/Compare To Constant  relop=>  const=0.01  OutDataTypeStr=boolean
  Counter Free-Running : simulink/Sources/Counter Free-Running  NumBits=32  tsamp=-1
  Data Type Conversion{,1..2,4} (4 alike) : DataTypeConversion  OutDataTypeStr=uint8  RndMeth=Nearest
  Delay One Step : Delay  DelayLength=1
  Demux : Demux  Outputs=3
  Difference between sonar and pressure : Sum  Inputs=+-
  Gain : Gain  Gain=Estimator.pos.visDeltaXYMax
  Gain1 : Gain  Gain=Estimator.pos.visDeltaXYMax
  Geofencing error : Subsystem  TreatAsAtomicUnit=on
  GreaterThan : RelationalOperator  Operator=>  OutDataTypeStr=boolean  RndMeth=Simplest
  "GreaterThan  " : RelationalOperator  Operator=>  OutDataTypeStr=boolean  RndMeth=Simplest
  If : If  NumInputs=4  ElseIfExpressions=u2 > 0, u3> 0,u4>0
  Logical Operator : Logic  Operator=OR  AllPortsSameDT=off
  Logical Operator1 : Logic  AllPortsSameDT=off  OutDataTypeStr=boolean
  Logical Operator2 : Logic  AllPortsSameDT=off  OutDataTypeStr=boolean
  Logical Operator3 : Logic  Operator=OR  AllPortsSameDT=off
  Merge : Merge  Inputs=5  InitialOutput=0
  "No optical flow " : Subsystem  TreatAsAtomicUnit=on
  Normal condition : Subsystem  TreatAsAtomicUnit=on
  Subtract : Sum  Inputs=-+
  Subtract1 : Sum  Inputs=-+
  Switch : Switch  Criteria=u2 > Threshold
  Ultrasound improper : Subsystem  TreatAsAtomicUnit=on
  Wait  3 Seconds : Constant  Value=200*3
  estimator/Optical flow error : Subsystem  TreatAsAtomicUnit=on
  states_estim1 : InportShadow
  Flag : Outport
  wires:
  Bus Selector4/1 -> Abs/1  "<X>"
  states_estim/1 -> Bus Selector4/1
  Bus Selector4/2 -> Abs1/1  "<Y>"
  Compare To Constant/1 -> Logical Operator/1
  Compare To Constant1/1 -> Logical Operator/2
  Abs/1 -> Compare To Constant/1
  Abs1/1 -> Compare To Constant1/1
  Logical Operator/1 -> Data Type Conversion/1
  Bus Selector/1 -> Demux/1  "<opticalFlow_data>"
  Demux/1 -> Abs4/1, Gain/1  "dx_OF"
  Demux/2 -> Gain1/1, Abs5/1  "dy_OF"
  Bus Selector4/3 -> Subtract/1  "<dx>"
  Subtract/1 -> Abs2/1
  Subtract1/1 -> Abs3/1
  Abs2/1 -> Compare To Constant2/1
  Abs3/1 -> Compare To Constant3/1
  Compare To Constant5/1 -> Logical Operator2/2
  Abs4/1 -> Compare To Constant4/1
  Abs5/1 -> Compare To Constant5/1
  Compare To Constant3/1 -> Logical Operator2/1
  Logical Operator1/1 -> Logical Operator3/1
  Logical Operator2/1 -> Logical Operator3/2
  Logical Operator3/1 -> Data Type Conversion1/1
  Gain/1 -> Subtract/2
  Bus Selector4/4 -> Subtract1/1  "<dy>"
  Gain1/1 -> Subtract1/2
  Compare To Constant4/1 -> Logical Operator1/1
  Compare To Constant2/1 -> Logical Operator1/2
  Sensors/1 -> Bus Selector1/1
  Bus Selector1/1 -> Bus Selector/1  "<VisionSensors>"
  Merge/1 -> Flag/1
  If/1 -> Geofencing error/Action
  If/2 -> estimator/Optical flow error/Action
  If/5 -> Normal condition/Action
  Geofencing error/1(Out1) -> Merge/1
  estimator/Optical flow error/1(Out1) -> Merge/2
  Normal condition/1(Out1) -> Merge/5
  Data Type Conversion/1 -> If/1
  Data Type Conversion1/1 -> If/2
  Check error condition/1 -> "   "/1
  Demux/3 -> Switch/1  "OF_status"
  Delay One Step/1 -> "  "/2
  Add/1 -> Delay One Step/1, "50 continuous OF errors "/1
  "  "/1 -> Add/2
  "50 continuous OF errors "/1 -> Data Type Conversion2/1
  Data Type Conversion2/1 -> If/3
  "No optical flow "/1(Out1) -> Merge/3
  If/3 -> "No optical flow "/Action
  "   "/1 -> Add/1, "  "/1
  Counter Free-Running/1 -> GreaterThan/1
  Wait  3 Seconds/1 -> GreaterThan/2
  Switch/1 -> Check error condition/1
  " "/1 -> Switch/3
  "    "/1 -> "         "/3
  Difference between sonar and pressure/1 -> "         "/1
  Bus Selector2/1 -> Difference between sonar and pressure/1  "<Z>"
  GreaterThan/1 -> Switch/2, "         "/2
  "         "/1 -> "Abs  "/1
  "Abs  "/1 -> "GreaterThan  "/1
  0.5 meters/1 -> "GreaterThan  "/2
  Alt_prs/1 -> Difference between sonar and pressure/2
  "GreaterThan  "/1 -> Data Type Conversion4/1
  states_estim1/1 -> Bus Selector2/1
  Data Type Conversion4/1 -> If/4
  Ultrasound improper/1(Out1) -> Merge/4
  If/4 -> Ultrasound improper/Action

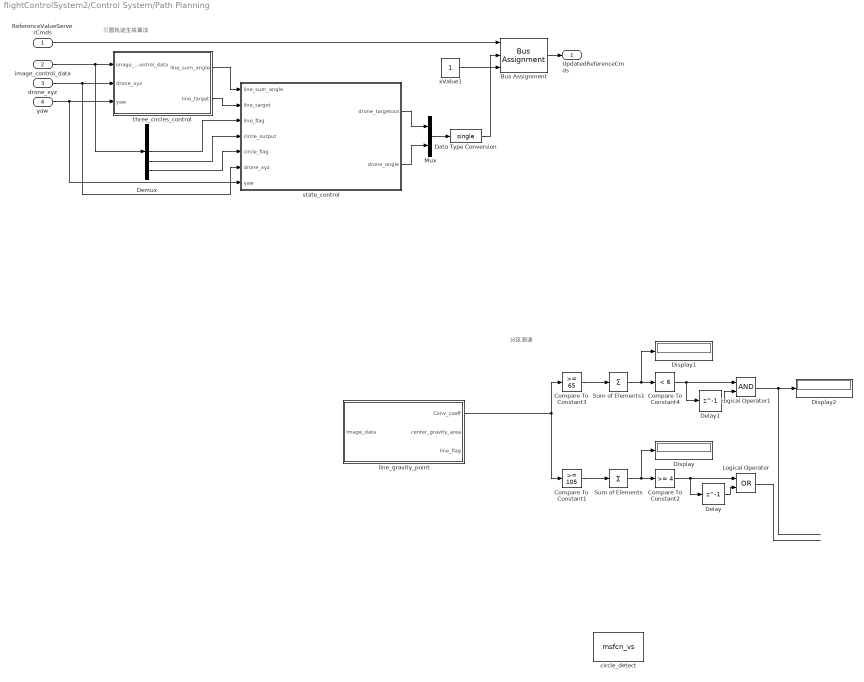
== system flightControlSystem2/Control System/Path Planning ==
  note: 三圆轨迹生成算法
  note: 分区测速
  ReferenceValueServerCmds : Inport
  image_control_data : Inport  Port=2
  drone_xyz : Inport  Port=3
  yaw : Inport  Port=4
  Bus Assignment : BusAssignment  AssignedSignals=pos_ref,takeoff_flag
  Compare To Constant1 : simulink/Logic and Bit Operations/Compare To Constant  relop=>=  const=105  OutDataTypeStr=boolean
  Compare To Constant2 : simulink/Logic and Bit Operations/Compare To Constant  relop=>=  const=4  OutDataTypeStr=boolean
  Compare To Constant3 : simulink/Logic and Bit Operations/Compare To Constant  relop=>=  const=65  OutDataTypeStr=boolean
  Compare To Constant4 : simulink/Logic and Bit Operations/Compare To Constant  relop=<  const=6  OutDataTypeStr=boolean
  Data Type Conversion : DataTypeConversion  OutDataTypeStr=single
  Delay : Delay  DelayLength=1  InitialCondition=0
  Delay1 : Delay  DelayLength=1  InitialCondition=0
  Demux : Demux  Outputs=5
  Display : Display
  Display1 : Display
  Display2 : Display
  Logical Operator : Logic  Operator=OR  AllPortsSameDT=off  OutDataTypeStr=boolean
  Logical Operator1 : Logic  AllPortsSameDT=off  OutDataTypeStr=boolean
  Mux : Mux  Inputs=2
  Sum of Elements : Sum  Inputs=+  OutDataTypeStr=int8
  Sum of Elements1 : Sum  Inputs=+  OutDataTypeStr=int8
  circle_detect : M-S-Function  FunctionName=msfcn_vs
      mask Display: disp('dt           = u(2)\ny(t + dt) = u(t)')
  line_gravity_point : MATLAB Function  TreatAsAtomicUnit=on
  state_control : MATLAB Function  TreatAsAtomicUnit=on
  three_circles_control : MATLAB Function  TreatAsAtomicUnit=on
  xValue1 : Constant  OutDataTypeStr=boolean
  UpdatedReferenceCmds : Outport
  wires:
  ReferenceValueServerCmds/1 -> Bus Assignment/1
  Data Type Conversion/1 -> Bus Assignment/2
  Bus Assignment/1 -> UpdatedReferenceCmds/1
  xValue1/1 -> Bus Assignment/3
  Logical Operator/1 -> ?
  Sum of Elements/1 -> Compare To Constant2/1, Display/1
  three_circles_control/2(line_target) -> state_control/2(line_target)
  Delay1/1 -> Logical Operator1/2
  Logical Operator1/1 -> Display2/1
  Compare To Constant1/1 -> Sum of Elements/1
  Compare To Constant2/1 -> Logical Operator/1, Delay/1
  Compare To Constant4/1 -> Delay1/1, Logical Operator1/1
  Compare To Constant3/1 -> Sum of Elements1/1
  Delay/1 -> Logical Operator/2
  Sum of Elements1/1 -> Compare To Constant4/1, Display1/1
  three_circles_control/1(line_sum_angle) -> state_control/1(line_sum_angle)
  line_gravity_point/1(Conv_coeff) -> Compare To Constant1/1, Compare To Constant3/1
  image_control_data/1 -> Demux/1, three_circles_control/1(image_control_data)
  drone_xyz/1 -> three_circles_control/2(drone_xyz), state_control/6(drone_xyz)
  yaw/1 -> three_circles_control/3(yaw), state_control/7(yaw)
  Demux/3 -> state_control/3(line_flag)
  Demux/4 -> state_control/4(circle_output)
  Demux/5 -> state_control/5(circle_flag)
  state_control/1(drone_targetout) -> Mux/1
  state_control/2(drone_angle) -> Mux/2
  Mux/1 -> Data Type Conversion/1

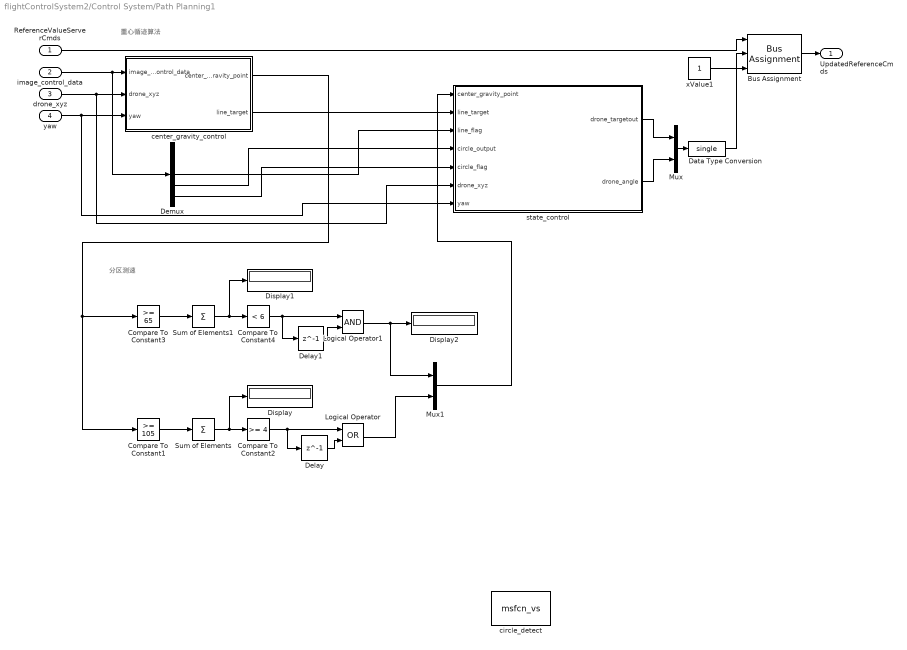
== system flightControlSystem2/Control System/Path Planning1 ==
  note: 重心循迹算法
  note: 分区测速
  ReferenceValueServerCmds : Inport
  image_control_data : Inport  Port=2
  drone_xyz : Inport  Port=3
  yaw : Inport  Port=4
  Bus Assignment : BusAssignment  AssignedSignals=pos_ref,takeoff_flag
  Compare To Constant1 : simulink/Logic and Bit Operations/Compare To Constant  relop=>=  const=105  OutDataTypeStr=boolean
  Compare To Constant2 : simulink/Logic and Bit Operations/Compare To Constant  relop=>=  const=4  OutDataTypeStr=boolean
  Compare To Constant3 : simulink/Logic and Bit Operations/Compare To Constant  relop=>=  const=65  OutDataTypeStr=boolean
  Compare To Constant4 : simulink/Logic and Bit Operations/Compare To Constant  relop=<  const=6  OutDataTypeStr=boolean
  Data Type Conversion : DataTypeConversion  OutDataTypeStr=single
  Delay : Delay  DelayLength=1  InitialCondition=0
  Delay1 : Delay  DelayLength=1  InitialCondition=0
  Demux : Demux  Outputs=5
  Display : Display
  Display1 : Display
  Display2 : Display
  Logical Operator : Logic  Operator=OR  AllPortsSameDT=off  OutDataTypeStr=boolean
  Logical Operator1 : Logic  AllPortsSameDT=off  OutDataTypeStr=boolean
  Mux : Mux  Inputs=2
  Mux1 : Mux  Inputs=2
  Sum of Elements : Sum  Inputs=+  OutDataTypeStr=int8
  Sum of Elements1 : Sum  Inputs=+  OutDataTypeStr=int8
  center_gravity_control : MATLAB Function  TreatAsAtomicUnit=on
  circle_detect : M-S-Function  FunctionName=msfcn_vs
      mask Display: disp('dt           = u(2)\ny(t + dt) = u(t)')
  state_control : MATLAB Function  TreatAsAtomicUnit=on
  xValue1 : Constant  OutDataTypeStr=boolean
  UpdatedReferenceCmds : Outport
  wires:
  ReferenceValueServerCmds/1 -> Bus Assignment/1
  Data Type Conversion/1 -> Bus Assignment/2
  Bus Assignment/1 -> UpdatedReferenceCmds/1
  xValue1/1 -> Bus Assignment/3
  Logical Operator/1 -> Mux1/2
  Sum of Elements/1 -> Compare To Constant2/1, Display/1
  center_gravity_control/2(line_target) -> state_control/2(line_target)
  Delay1/1 -> Logical Operator1/2
  Compare To Constant1/1 -> Sum of Elements/1
  Compare To Constant2/1 -> Logical Operator/1, Delay/1
  Compare To Constant4/1 -> Delay1/1, Logical Operator1/1
  Compare To Constant3/1 -> Sum of Elements1/1
  Delay/1 -> Logical Operator/2
  Sum of Elements1/1 -> Compare To Constant4/1, Display1/1
  image_control_data/1 -> Demux/1, center_gravity_control/1(image_control_data)
  drone_xyz/1 -> center_gravity_control/2(drone_xyz), state_control/6(drone_xyz)
  yaw/1 -> center_gravity_control/3(yaw), state_control/7(yaw)
  Demux/3 -> state_control/3(line_flag)
  Demux/4 -> state_control/4(circle_output)
  Demux/5 -> state_control/5(circle_flag)
  state_control/1(drone_targetout) -> Mux/1
  state_control/2(drone_angle) -> Mux/2
  Mux/1 -> Data Type Conversion/1
  center_gravity_control/1(center_gravity_point) -> Compare To Constant1/1, Compare To Constant3/1
  Logical Operator1/1 -> Mux1/1, Display2/1
  Mux1/1 -> state_control/1(center_gravity_point)

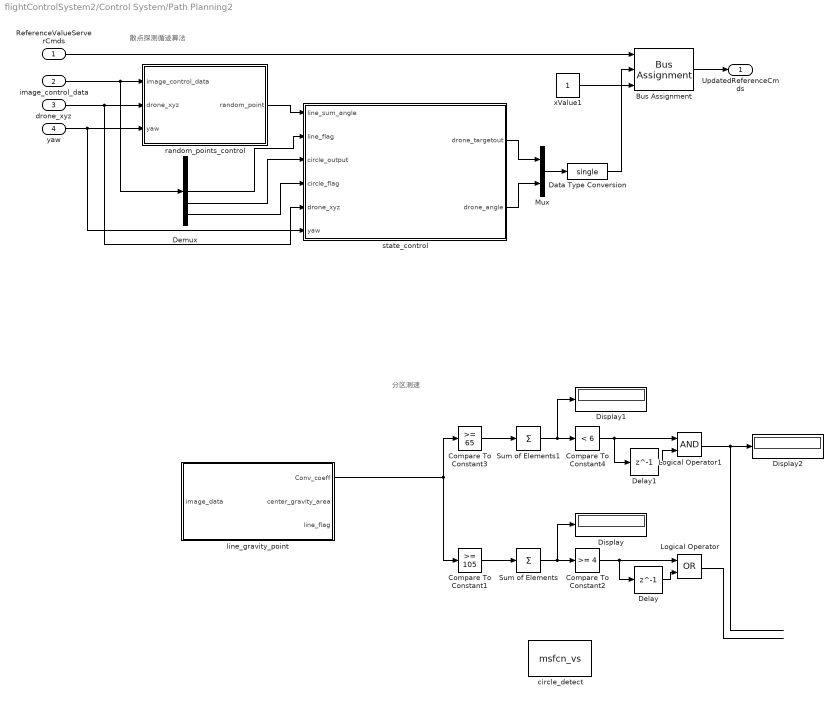
== system flightControlSystem2/Control System/Path Planning2 ==
  note: 散点探测循迹算法
  note: 分区测速
  ReferenceValueServerCmds : Inport
  image_control_data : Inport  Port=2
  drone_xyz : Inport  Port=3
  yaw : Inport  Port=4
  Bus Assignment : BusAssignment  AssignedSignals=pos_ref,takeoff_flag
  Compare To Constant1 : simulink/Logic and Bit Operations/Compare To Constant  relop=>=  const=105  OutDataTypeStr=boolean
  Compare To Constant2 : simulink/Logic and Bit Operations/Compare To Constant  relop=>=  const=4  OutDataTypeStr=boolean
  Compare To Constant3 : simulink/Logic and Bit Operations/Compare To Constant  relop=>=  const=65  OutDataTypeStr=boolean
  Compare To Constant4 : simulink/Logic and Bit Operations/Compare To Constant  relop=<  const=6  OutDataTypeStr=boolean
  Data Type Conversion : DataTypeConversion  OutDataTypeStr=single
  Delay : Delay  DelayLength=1  InitialCondition=0
  Delay1 : Delay  DelayLength=1  InitialCondition=0
  Demux : Demux  Outputs=5
  Display : Display
  Display1 : Display
  Display2 : Display
  Logical Operator : Logic  Operator=OR  AllPortsSameDT=off  OutDataTypeStr=boolean
  Logical Operator1 : Logic  AllPortsSameDT=off  OutDataTypeStr=boolean
  Mux : Mux  Inputs=2
  Sum of Elements : Sum  Inputs=+  OutDataTypeStr=int8
  Sum of Elements1 : Sum  Inputs=+  OutDataTypeStr=int8
  circle_detect : M-S-Function  FunctionName=msfcn_vs
      mask Display: disp('dt           = u(2)\ny(t + dt) = u(t)')
  line_gravity_point : MATLAB Function  TreatAsAtomicUnit=on
  random_points_control : MATLAB Function  TreatAsAtomicUnit=on
  state_control : MATLAB Function  TreatAsAtomicUnit=on
  xValue1 : Constant  OutDataTypeStr=boolean
  UpdatedReferenceCmds : Outport
  wires:
  ReferenceValueServerCmds/1 -> Bus Assignment/1
  Data Type Conversion/1 -> Bus Assignment/2
  Bus Assignment/1 -> UpdatedReferenceCmds/1
  xValue1/1 -> Bus Assignment/3
  Logical Operator/1 -> ?
  Sum of Elements/1 -> Compare To Constant2/1, Display/1
  Delay1/1 -> Logical Operator1/2
  Logical Operator1/1 -> Display2/1
  Compare To Constant1/1 -> Sum of Elements/1
  Compare To Constant2/1 -> Logical Operator/1, Delay/1
  Compare To Constant4/1 -> Delay1/1, Logical Operator1/1
  Compare To Constant3/1 -> Sum of Elements1/1
  Delay/1 -> Logical Operator/2
  Sum of Elements1/1 -> Compare To Constant4/1, Display1/1
  random_points_control/1(random_point) -> state_control/1(line_sum_angle)
  line_gravity_point/1(Conv_coeff) -> Compare To Constant1/1, Compare To Constant3/1
  image_control_data/1 -> Demux/1, random_points_control/1(image_control_data)
  drone_xyz/1 -> random_points_control/2(drone_xyz), state_control/5(drone_xyz)
  yaw/1 -> random_points_control/3(yaw), state_control/6(yaw)
  Demux/3 -> state_control/2(line_flag)
  Demux/4 -> state_control/3(circle_output)
  Demux/5 -> state_control/4(circle_flag)
  state_control/1(drone_targetout) -> Mux/1
  state_control/2(drone_angle) -> Mux/2
  Mux/1 -> Data Type Conversion/1
